simulink model "R3GDL"  (Simulink 9.0)
settings: Solver=ode45  StartTime=0.0  StopTime=Tsim  MaxStep=1e-3  RelTol=1e-3  EnableMultiTasking=on
values from neighbouring files (symbols this model uses):
  A_a = [2    1.5  0.5]    [excitacion.m]
  A_b = [7    4   3]    [excitacion.m]
  Im_cc = [0  0.4  0.15]    [excitacion.m]
  R1 = 50    [M_def_pos.m]    (also in MinimosCuadrados.m; ModeloDinamico_R3GDL.m)
  R2 = 30    [M_def_pos.m]    (also in MinimosCuadrados.m; ModeloDinamico_R3GDL.m)
  R3 = 15    [M_def_pos.m]    (also in MinimosCuadrados.m; ModeloDinamico_R3GDL.m)
  tau = 1/wc*tan(70*pi/180)    [Controladores.m]    (also in excitacion.m = 8)
  tau2 = 3    [excitacion.m]
  Ts = 1e-3    (= 0.001)    [excitacion.m]
  W_a = [0.5  0.5  0.5]*2*pi    [excitacion.m]
  W_b = [3.5 2.5  2.5]*2*pi    [excitacion.m]
settings Model: Creator=mortega  LastModifiedBy=Alvaro  ExtModeTrigMode=oneshot  ExtModeArmWhenConnect=off
settings DataIOCC: SignalLoggingSaveFormat=ModelDataLogs
settings OptimizationCC: BlockReduction=off  BooleanDataType=off  ExpressionDepthLimit=2147483647  InitFltsAndDblsToZero=on
settings DebuggingCC: SaveWithParameterizedLinksMsg=none  SignalResolutionControl=TryResolveAllWithWarning  MultiTaskDSMMsg=warning  MultiTaskCondExecSysMsg=none  FcnCallInpInsideContextMsg=warning  StateNameClashWarn=warning  StrictBusMsg=None
settings HardwareCC: TargetUnknown=on
settings GRTTargetCC: TargetFcnLib=ansi_tfl_tmw.mat  CombineOutputUpdateFcns=off  GRTInterface=on

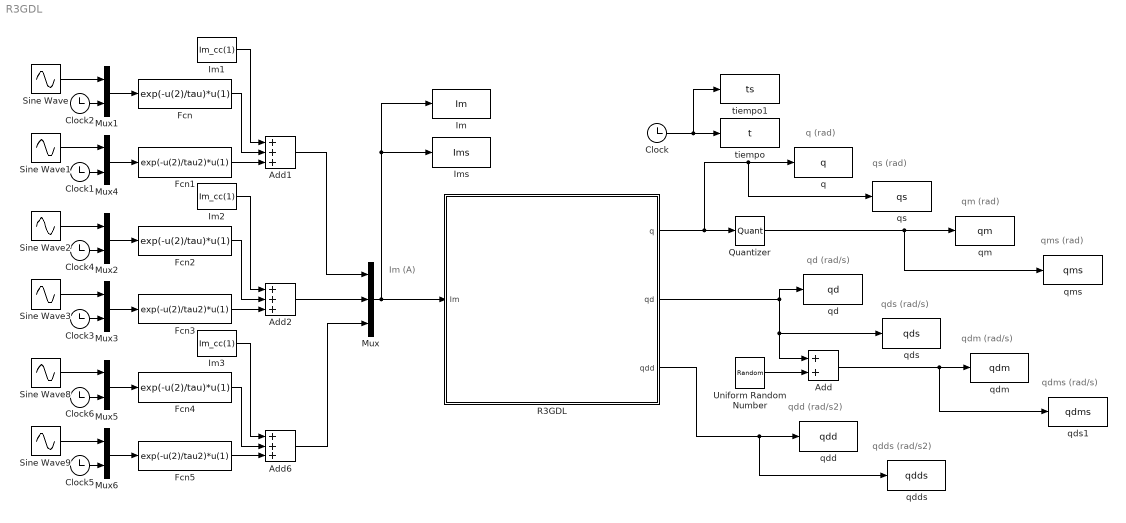
== system R3GDL ==
  note: Im (A)
  note: q (rad)
  note: qd (rad/s)
  note: qdd (rad/s2)
  note: qs (rad)
  note: qds (rad/s)
  note: qdds (rad/s2)
  note: qm (rad)
  note: qms (rad)
  note: qdm (rad/s)
  note: qdms (rad/s)
  Add : Sum
  Add1 : Sum  Inputs=+++
  Add2 : Sum  Inputs=+++
  Add6 : Sum  Inputs=+++
  Clock{,1..6} (7 alike) : Clock
  Fcn : Fcn  Expr=exp(-u(2)/tau)*u(1)
  Fcn1 : Fcn  Expr=exp(-u(2)/tau2)*u(1)
  Fcn2 : Fcn  Expr=exp(-u(2)/tau)*u(1)
  Fcn3 : Fcn  Expr=exp(-u(2)/tau2)*u(1)
  Fcn4 : Fcn  Expr=exp(-u(2)/tau)*u(1)
  Fcn5 : Fcn  Expr=exp(-u(2)/tau2)*u(1)
  Im : ToWorkspace  VariableName=Im  SampleTime=-1
  Im1 : Constant  Value=Im_cc(1)
  Im2 : Constant  Value=Im_cc(1)
  Im3 : Constant  Value=Im_cc(1)
  Ims : ToWorkspace  VariableName=Ims  SampleTime=Ts
  Mux : Mux  Inputs=3
  Mux{1..6} (6 alike) : Mux  Inputs=2
  Quantizer : Quantizer  QuantizationInterval=2*pi/512./[R1 R2 R3]
  R3GDL : Subsystem  mask(Control y Programación de Robots (4 GIERM)){NGrupo=3, q1_ini=0, q2_ini=0, q3_ini=0, Bl_q1=off, Bl_q2=off, Bl_q3=off, AccionamientoDirecto=off}
      mask prompts: NGrupo "Nº de GRUPO"; q1_ini "q1 inicial  (rad)"; q2_ini "q2 inicial (rad)"; q3_ini "q3_inicial (rad)"; Bl_q1 "Bloqueo q1"; Bl_q2 "Bloqueo q2"; Bl_q3 "Bloqueo q3"; AccionamientoDirecto "Accionamiento directo"
      mask help: Robot de 3 grados de libertad RRR
      mask Display:
      | image(imread('R3GDL_RRR.JPG'));
      | port_label('output', 1, 'q');
      | port_label('output', 2, 'qd');
      | port_label('output', 3, 'qdd');
      | port_label('input', 1, 'Im')
  Sine Wave : Sin  Amplitude=A_a(1)  Frequency=W_a(1)  SampleTime=0
  Sine Wave1 : Sin  Amplitude=A_b(1)  Frequency=W_b(1)  SampleTime=0
  Sine Wave2 : Sin  Amplitude=A_a(2)  Frequency=W_a(2)  SampleTime=0
  Sine Wave3 : Sin  Amplitude=A_b(2)  Frequency=W_b(2)  SampleTime=0
  Sine Wave8 : Sin  Amplitude=A_a(3)  Frequency=W_a(3)  SampleTime=0
  Sine Wave9 : Sin  Amplitude=A_b(3)  Frequency=W_b(3)  SampleTime=0
  Uniform Random Number : UniformRandomNumber  Minimum=-1500*2*pi/60./[R1 R2 R3]*0.02  Maximum=1500*2*pi/60./[R1 R2 R3]*0.02  SampleTime=Ts/10
  q : ToWorkspace  VariableName=q  SampleTime=-1
  qd : ToWorkspace  VariableName=qd  SampleTime=-1
  qdd : ToWorkspace  VariableName=qdd  SampleTime=-1
  qdds : ToWorkspace  VariableName=qdds  SampleTime=Ts
  qdm : ToWorkspace  VariableName=qdm  SampleTime=-1
  qds : ToWorkspace  VariableName=qds  SampleTime=Ts
  qds1 : ToWorkspace  VariableName=qdms  SampleTime=Ts
  qm : ToWorkspace  VariableName=qm  SampleTime=-1
  qms : ToWorkspace  VariableName=qms  SampleTime=Ts
  qs : ToWorkspace  VariableName=qs  SampleTime=Ts
  tiempo : ToWorkspace  VariableName=t  SampleTime=-1
  tiempo1 : ToWorkspace  VariableName=ts  SampleTime=Ts
  wires:
  Clock/1 -> tiempo1/1, tiempo/1
  Add/1 -> qdm/1, qds1/1
  Uniform Random Number/1 -> Add/2
  Quantizer/1 -> qm/1, qms/1
  R3GDL/3(qdd) -> qdd/1, qdds/1
  R3GDL/2(qd) -> qds/1, Add/1, qd/1
  R3GDL/1(q) -> Quantizer/1, q/1, qs/1
  Mux/1 -> Ims/1, Im/1, R3GDL/1(Im)
  Mux1/1 -> Fcn/1
  Im1/1 -> Add1/1
  Clock2/1 -> Mux1/2
  Fcn/1 -> Add1/2
  Add1/1 -> Mux/1
  Mux4/1 -> Fcn1/1
  Fcn1/1 -> Add1/3
  Clock1/1 -> Mux4/2
  Clock3/1 -> Mux3/2
  Fcn3/1 -> Add2/3
  Mux3/1 -> Fcn3/1
  Fcn2/1 -> Add2/2
  Clock4/1 -> Mux2/2
  Im2/1 -> Add2/1
  Mux2/1 -> Fcn2/1
  Add2/1 -> Mux/2
  Mux5/1 -> Fcn4/1
  Im3/1 -> Add6/1
  Clock6/1 -> Mux5/2
  Fcn4/1 -> Add6/2
  Mux6/1 -> Fcn5/1
  Fcn5/1 -> Add6/3
  Clock5/1 -> Mux6/2
  Add6/1 -> Mux/3
  Sine Wave/1 -> Mux1/1
  Sine Wave1/1 -> Mux4/1
  Sine Wave2/1 -> Mux2/1
  Sine Wave3/1 -> Mux3/1
  Sine Wave8/1 -> Mux5/1
  Sine Wave9/1 -> Mux6/1

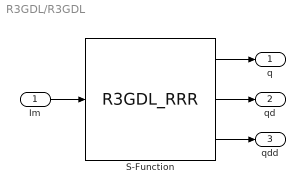
== system R3GDL/R3GDL ==
  Im : Inport
  S-Function : S-Function  FunctionName=R3GDL_RRR  Parameters=[q1_ini; q2_ini; q3_ini]; [Bl_q1; Bl_q2; Bl_q3]; AccionamientoDirecto; NGrupo  SFunctionDeploymentMode=off  EnableBusSupport=off
  q : Outport
  qd : Outport  Port=2
  qdd : Outport  Port=3
  wires:
  Im/1 -> S-Function/1
  S-Function/1 -> q/1
  S-Function/2 -> qd/1
  S-Function/3 -> qdd/1
